simulink model "task2_4"  (R2023a)
settings: Solver=VariableStepAuto  StartTime=0.0  StopTime=10.0  RelTol=1e-8
settings Model: Creator=user  LastModifiedBy=user

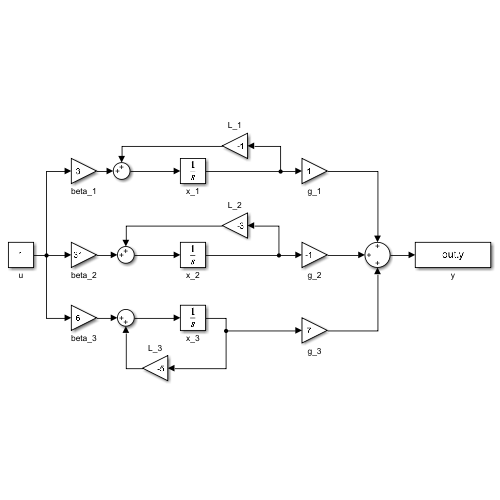
[thumbnail: Simulink's stored preview of the top-level diagram]
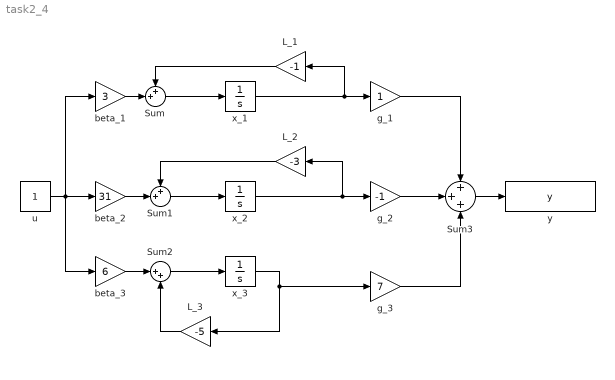
== system task2_4 ==
  L_1 : Gain  Gain=-1
  L_2 : Gain  Gain=-3
  L_3 : Gain  Gain=-5
  Sum : Sum  Inputs=++|
  Sum1 : Sum  Inputs=++|
  Sum2 : Sum  Inputs=|++
  Sum3 : Sum  Inputs=+++
  beta_1 : Gain  Gain=3
  beta_2 : Gain  Gain=31
  beta_3 : Gain  Gain=6
  g_1 : Gain
  g_2 : Gain  Gain=-1
  g_3 : Gain  Gain=7
  u : Constant
  x_1 : Integrator
  x_2 : Integrator
  x_3 : Integrator
  y : ToWorkspace  VariableName=y  SaveFormat=Timeseries  SampleTime=-1
  wires:
  u/1 -> beta_3/1, beta_1/1, beta_2/1
  beta_1/1 -> Sum/2
  Sum/1 -> x_1/1
  x_1/1 -> L_1/1, g_1/1
  L_1/1 -> Sum/1
  beta_2/1 -> Sum1/2
  Sum1/1 -> x_2/1
  x_2/1 -> g_2/1, L_2/1
  L_2/1 -> Sum1/1
  beta_3/1 -> Sum2/1
  Sum2/1 -> x_3/1
  x_3/1 -> L_3/1, g_3/1
  L_3/1 -> Sum2/2
  Sum3/1 -> y/1
  g_1/1 -> Sum3/1
  g_2/1 -> Sum3/2
  g_3/1 -> Sum3/3
